simulink model "TEST_magnetics"  (R2019b)
settings: Solver=VariableStepAuto  StartTime=0.0  StopTime=inf  RelTol=1e-3
undefined symbols (not defined in the file or in its folder): ALGO_SET
libraries: aerolibgravity2 x1
settings Model: Creator=sl  LastModifiedBy=sl

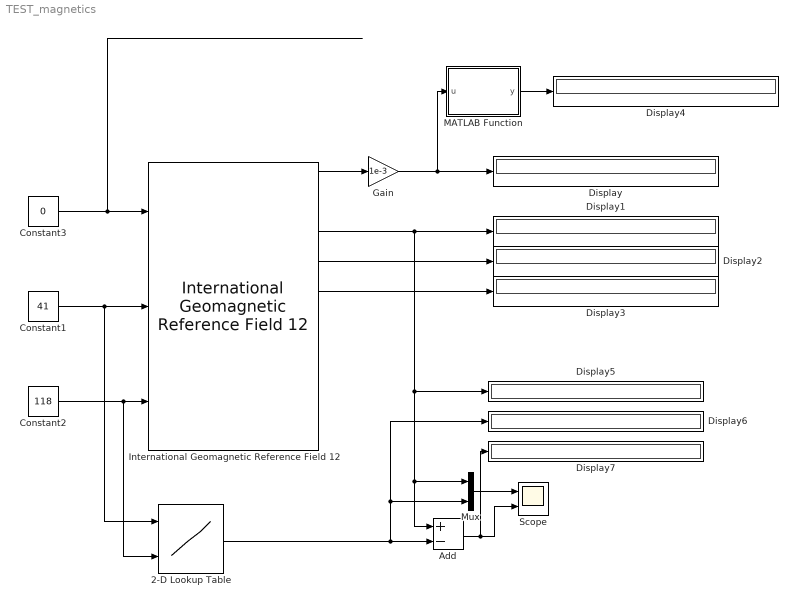
== system TEST_magnetics ==
  2-D Lookup Table : Lookup_n-D  BreakpointsForDimension1=ALGO_SET.magneticData.lat  BreakpointsForDimension2=ALGO_SET.magneticData.lon  Table=ALGO_SET.magneticData.magDec  ExtrapMethod=Clip  UseLastTableValue=on  InternalRulePriority=Speed  RndMeth=Simplest  InputSameDT=on
  Add : Sum  Inputs=+-
  Constant1 : Constant  Value=41
  Constant2 : Constant  Value=118
  Constant3 : Constant  Value=0
  Display{,1..7} (8 alike) : Display
  Gain : Gain  Gain=1e-3
  International Geomagnetic Reference Field 12 : aerolibgravity2/International Geomagnetic Reference Field 12  units=Metric (MKS)  time_in=off  month=January  day=1  year=2020  action=None  sv_out=on
      settings: SourceProductName=Aerospace Blockset  SourceProductBaseCode=AE
  MATLAB Function : MATLAB Function  TreatAsAtomicUnit=on
  Mux : Mux  Inputs=2
  Scope : Scope  NumInputPorts=2
  wires:
  International Geomagnetic Reference Field 12/1 -> Gain/1
  International Geomagnetic Reference Field 12/3 -> Display1/1, Mux/1, Add/1, Display5/1
  International Geomagnetic Reference Field 12/4 -> Display2/1
  International Geomagnetic Reference Field 12/5 -> Display3/1
  Constant3/1 -> International Geomagnetic Reference Field 12/1
  Constant1/1 -> 2-D Lookup Table/1, International Geomagnetic Reference Field 12/2
  Constant2/1 -> 2-D Lookup Table/2, International Geomagnetic Reference Field 12/3
  Gain/1 -> MATLAB Function/1(u), Display/1
  MATLAB Function/1(y) -> Display4/1
  2-D Lookup Table/1 -> Display6/1, Mux/2, Add/2
  Add/1 -> Display7/1, Scope/2
  Mux/1 -> Scope/1

== matlab function TEST_magnetics/MATLAB Function ==
  data: u input; y output
function y = fcn(u)

y = norm(u);
